simulink model "PhaseCavitySim"  (R2017b)
settings: Solver=ode45  StartTime=0.0  StopTime=10e-6  MaxStep=5e-12  RelTol=1e-3  EnableMultiTasking=on
values from neighbouring files (symbols this model uses):
  Fadc = 351e6    (= 351000000)    [setupPhaseCavity.m]    (also in setupPhaseCavity2604.m)
  Fbp = Fcav, wbp = 2*pi*Fbp    [setupPhaseCavity.m]    (also in setupPhaseCavity2604.m)
  Fcav = 2600e6 - 5* 13e6/14    (= 2595357142.86)    [setupPhaseCavity.m]    (also in setupPhaseCavity2604.m)
  Fgun = 185.7143e6    (= 185714300)    [setupPhaseCavity.m]    (also in setupPhaseCavity2604.m)
  Fif = Fcav - Flo    (= 78928571.4286)    [setupPhaseCavity.m]    (also in setupPhaseCavity2604.m)
  Flo = 2*Frf - 5/21*Fadc    (= 2516428571.43)    [setupPhaseCavity.m]    (also in setupPhaseCavity2604.m)
  Flp = 1e9, wlp = 2 *pi*Flp    [setupPhaseCavity.m]    (also in setupPhaseCavity2604.m)
  Frf = 1300e6    (= 1300000000)    [setupPhaseCavity.m]    (also in setupPhaseCavity2604.m)
  Idark = 400e-9    (= 4e-07)    [setupPhaseCavity.m]    (also in setupPhaseCavity2604.m)
  qbeam = 100e-12    (= 1e-10)    [setupPhaseCavity.m]    (also in setupPhaseCavity2604.m)
  Qbp = 3    [setupPhaseCavity.m]    (also in setupPhaseCavity2604.m)
  Qcav = 6060    [setupPhaseCavity.m]    (also in setupPhaseCavity2604.m)
  Qif = 4.2    [setupPhaseCavity.m]    (also in setupPhaseCavity2604.m)
  wcav = 2*pi*Fcav    (= 16307109866.9)    [setupPhaseCavity.m]    (also in setupPhaseCavity2604.m)
  wif = 2*pi*Fif    (= 495922840.317)    [setupPhaseCavity.m]    (also in setupPhaseCavity2604.m)
undefined symbols (not defined in the file or in its folder): wbp, wlp
settings Model: Creator=ssmith  LastModifiedBy=ssmith
settings DataIOCC: LimitDataPoints=on  SaveFormat=Array
settings OptimizationCC: ExpressionDepthLimit=2147483647  LifeSpan=inf
settings DebuggingCC: UnderspecifiedInitializationDetection=Classic  MergeDetectMultiDrivingBlocksExec=none  SolverPrmCheckMsg=warning  StateNameClashWarn=warning  SFUnexpectedBacktrackingDiag=warning  SFNoUnconditionalDefaultTransitionDiag=warning  SFExecutionAtInitializationDiag=none
settings HardwareCC: ProdBitPerPointer=32  ProdBitPerSizeT=32  ProdBitPerPtrDiffT=32  ProdLargestAtomicFloat=None  ProdIntDivRoundTo=Undefined  ProdEndianess=Unspecified  ProdWordSize=32  ProdHWDeviceType=32-bit Generic
settings ModelReferenceCC: PropagateSignalLabelsOutOfModel=off
settings CodeAppCC: StateflowObjectComments=on
settings GRTTargetCC: TargetLangStandard=C89/C90 (ANSI)  GeneratePreprocessorConditionals=Disable all
settings ConfigComp: CovMetricSettings=dw  CovHtmlReporting=on  CovSaveCumulativeToWorkspaceVar=on  CovSaveSingleToWorkspaceVar=on  CovExternalEMLEnable=off

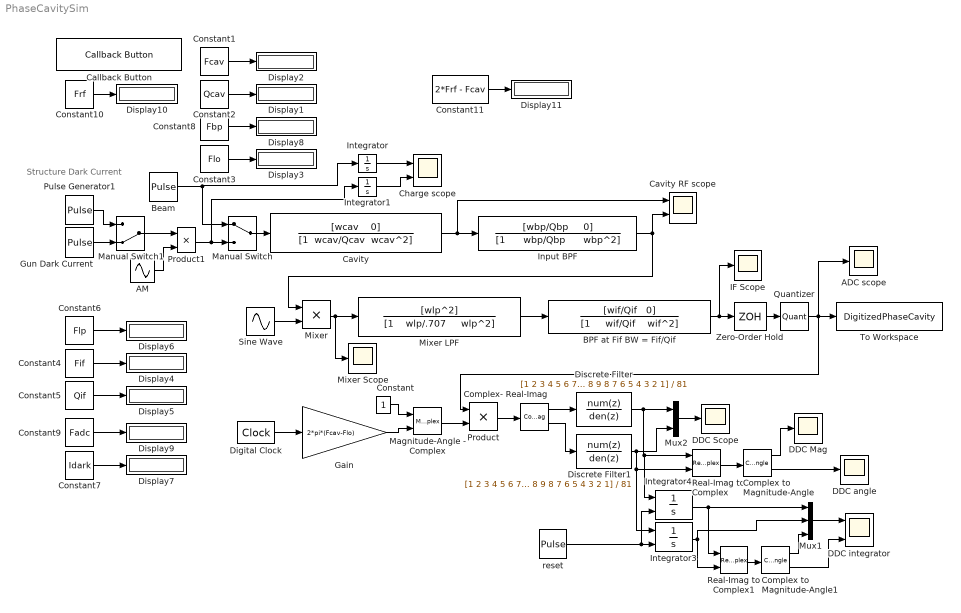
== system PhaseCavitySim ==
  note: Structure Dark Current
  ADC scope : Scope
  "AM " : Sin  Bias=1  Frequency=2*pi*abs( 2*Frf - Fcav)  SampleTime=0
  BPF at Fif BW = Fif/Qif : TransferFcn  Numerator="[wif/Qif   0]"  Denominator="[1     wif/Qif    wif^2]"
  Beam : DiscretePulseGenerator  PulseType=Time based  Amplitude=qbeam*Frf *100  Period=1  PulseWidth=1/Frf  PhaseDelay=20e-9
  Callback Button : CallbackButton  WebBlockId=103  ButtonText=setupPhaseCavity.m  PressDelay=500  RepeatInterval=0
      settings: ClickFcn=|
      | display('setting up phase cavity simulation parameters')
      | setupPhaseCavity
  Cavity : TransferFcn  Numerator="[wcav    0]"  Denominator="[1  wcav/Qcav  wcav^2]"
  Cavity RF scope : Scope  NumInputPorts=2
  Charge scope : Scope  NumInputPorts=2
  Complex to Magnitude-Angle : ComplexToMagnitudeAngle
  Complex to Magnitude-Angle1 : ComplexToMagnitudeAngle
  Complex- Real-Imag : ComplexToRealImag
  Constant : Constant
  Constant1 : Constant  Value=Fcav
  Constant10 : Constant  Value=Frf
  Constant11 : Constant  Value=2*Frf - Fcav
  Constant2 : Constant  Value=Qcav
  Constant3 : Constant  Value=Flo
  Constant4 : Constant  Value=Fif
  Constant5 : Constant  Value=Qif
  Constant6 : Constant  Value=Flp
  Constant7 : Constant  Value=Idark
  Constant8 : Constant  Value=Fbp
  Constant9 : Constant  Value=Fadc
  DDC integrator : Scope  NumInputPorts=2
  DDC Mag : Scope
  DDC Scope : Scope
  DDC angle : Scope
  Digital Clock : DigitalClock  SampleTime=1/Fadc
  Discrete Filter : DiscreteFilter  Numerator=[1 2 3 4 5 6 7 8 9 8 7 6 5 4 3 2 1]  Denominator=81  SampleTime=1/Fadc  NumCoefDataTypeStr=int8  DenCoefDataTypeStr=int8  OutDataTypeStr=Inherit: Same as input
  Discrete Filter1 : DiscreteFilter  Numerator=[1 2 3 4 5 6 7 8 9 8 7 6 5 4 3 2 1]  Denominator=81  SampleTime=1/Fadc
  Display{1..11} (11 alike) : Display
  Gain : Gain  Gain=2*pi*(Fcav-Flo)
  Gun Dark Current : DiscretePulseGenerator  PulseType=Time based  Amplitude=Idark * 1000  Period=1/Fgun  PulseWidth=0.1
  IF Scope : Scope
  Input BPF : TransferFcn  Numerator="[wbp/Qbp     0]"  Denominator="[1      wbp/Qbp      wbp^2]"
  Integrator : Integrator
  Integrator1 : Integrator
  Integrator3 : Integrator  ExternalReset=either
  Integrator4 : Integrator  ExternalReset=either
  Magnitude-Angle - Complex : MagnitudeAngleToComplex
  Manual Switch : ManualSwitch
  Manual Switch1 : ManualSwitch  CurrentSetting=0
  Mixer : Product  RndMeth=Zero
  Mixer Scope : Scope
  Mixer LPF : TransferFcn  Numerator=[wlp^2]  Denominator="[1    wlp/.707     wlp^2]"
  Mux1 : Mux  Inputs=3
  Mux2 : Mux  Inputs=2
  Product : Product  RndMeth=Zero
  Product1 : Product
  Pulse Generator1 : DiscretePulseGenerator  PulseType=Time based  Amplitude=Idark * 20  Period=1/Frf  PulseWidth=5
  Quantizer : Quantizer  QuantizationInterval=2^-15
  Real-Imag to Complex : RealImagToComplex
  Real-Imag to Complex1 : RealImagToComplex
  Sine Wave : Sin  Frequency=2*pi*Flo  SampleTime=0
  To Workspace : ToWorkspace  VariableName=DigitizedPhaseCavity  SaveFormat=Timeseries  SampleTime=-1
  Zero-Order Hold : ZeroOrderHold  SampleTime=1/Fadc
  reset : DiscretePulseGenerator  PulseType=Time based  Period=2e-6  PulseWidth=50
  wires:
  Cavity/1 -> Cavity RF scope/1, Input BPF/1
  Input BPF/1 -> Cavity RF scope/2, Mixer/1
  Mixer/1 -> Mixer Scope/1, Mixer LPF/1
  Mixer LPF/1 -> BPF at Fif BW = Fif/Qif/1
  Sine Wave/1 -> Mixer/2
  Quantizer/1 -> To Workspace/1, Product/1, ADC scope/1
  BPF at Fif BW = Fif/Qif/1 -> Zero-Order Hold/1, IF Scope/1
  Constant/1 -> Magnitude-Angle - Complex/1
  Digital Clock/1 -> Gain/1
  Gain/1 -> Magnitude-Angle - Complex/2
  Magnitude-Angle - Complex/1 -> Product/2
  Product/1 -> Complex- Real-Imag/1
  Complex- Real-Imag/2 -> Discrete Filter1/1
  Mux2/1 -> DDC Scope/1
  Complex- Real-Imag/1 -> Discrete Filter/1
  Discrete Filter/1 -> Integrator4/1, Real-Imag to Complex/1, Mux2/1
  Discrete Filter1/1 -> Mux2/2, Integrator3/1, Real-Imag to Complex/2
  Real-Imag to Complex/1 -> Complex to Magnitude-Angle/1
  Complex to Magnitude-Angle/1 -> DDC Mag/1
  Complex to Magnitude-Angle/2 -> DDC angle/1
  Constant1/1 -> Display2/1
  Constant2/1 -> Display1/1
  Constant3/1 -> Display3/1
  Beam/1 -> Manual Switch/1, Integrator/1
  Manual Switch/1 -> Cavity/1
  Integrator/1 -> Charge scope/1
  Integrator1/1 -> Charge scope/2
  Constant4/1 -> Display4/1
  Constant5/1 -> Display5/1
  Constant6/1 -> Display6/1
  Constant7/1 -> Display7/1
  Constant8/1 -> Display8/1
  Zero-Order Hold/1 -> Quantizer/1
  Pulse Generator1/1 -> Manual Switch1/1
  Gun Dark Current/1 -> Manual Switch1/2
  Manual Switch1/1 -> Product1/1
  "AM "/1 -> Product1/2
  Product1/1 -> Manual Switch/2, Integrator1/1
  Constant9/1 -> Display9/1
  Constant10/1 -> Display10/1
  Real-Imag to Complex1/1 -> Complex to Magnitude-Angle1/1
  Integrator4/1 -> Real-Imag to Complex1/1, Mux1/1
  Integrator3/1 -> Mux1/2, Real-Imag to Complex1/2
  Mux1/1 -> DDC integrator/1
  Complex to Magnitude-Angle1/1 -> Mux1/3
  Complex to Magnitude-Angle1/2 -> DDC integrator/2
  reset/1 -> Integrator4/2, Integrator3/2
  Constant11/1 -> Display11/1
